simulink model "svpwm_test"  (R2020b)
settings: Solver=VariableStepAuto  StartTime=0.0  StopTime=0.02  RelTol=1e-3
libraries: powerlib_meascontrol x6
settings Model: Creator=Administrator  LastModifiedBy=Administrator

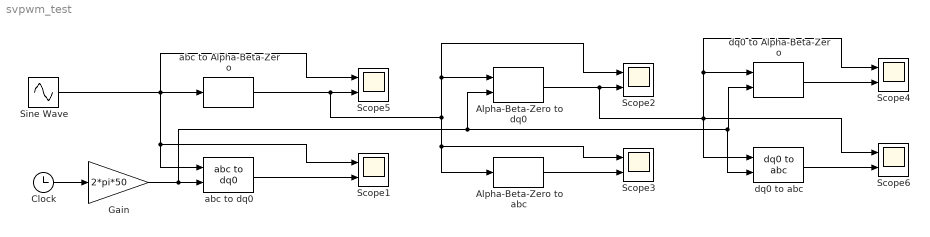
== system svpwm_test ==
  Alpha-Beta-Zero to abc : powerlib_meascontrol/Transformations/Alpha-Beta-Zero to abc
      settings: SourceProductBaseCode=PS
  Alpha-Beta-Zero to dq0 : powerlib_meascontrol/Transformations/Alpha-Beta-Zero to dq0  Alignment=90 degrees behind phase A axis
  Clock : Clock
  Gain : Gain  Gain=2*pi*50
  Scope{1..6} (6 alike) : Scope  NumInputPorts=2
  Sine Wave : Sin  Amplitude=100  Frequency=2*pi*50  Phase=[0 -2*pi/3 2*pi/3]  SampleTime=1e-6
  abc to Alpha-Beta-Zero : powerlib_meascontrol/Transformations/abc to Alpha-Beta-Zero
  abc to dq0 : powerlib_meascontrol/Transformations/abc to dq0  Alignment=90 degrees behind phase A axis
  dq0 to Alpha-Beta-Zero : powerlib_meascontrol/Transformations/dq0 to Alpha-Beta-Zero  Alignment=90 degrees behind phase A axis
      settings: SourceProductBaseCode=PS
  dq0 to abc : powerlib_meascontrol/Transformations/dq0 to abc  Alignment=90 degrees behind phase A axis
  wires:
  Sine Wave/1 -> abc to dq0/1, Scope1/1, Scope5/1, abc to Alpha-Beta-Zero/1
  abc to Alpha-Beta-Zero/1 -> Scope2/1, Alpha-Beta-Zero to dq0/1, Scope3/1, Alpha-Beta-Zero to abc/1, Scope5/2
  Gain/1 -> dq0 to abc/2, dq0 to Alpha-Beta-Zero/2, Alpha-Beta-Zero to dq0/2, abc to dq0/2
  Clock/1 -> Gain/1
  abc to dq0/1 -> Scope1/2
  Alpha-Beta-Zero to dq0/1 -> dq0 to abc/1, Scope6/1, Scope4/1, dq0 to Alpha-Beta-Zero/1, Scope2/2
  Alpha-Beta-Zero to abc/1 -> Scope3/2
  dq0 to Alpha-Beta-Zero/1 -> Scope4/2
  dq0 to abc/1 -> Scope6/2
